simulink subsystem "dL2dz"  (R2024a)
settings: Solver=VariableStepAuto  StartTime=0.0  StopTime=10.0  RelTol=1e-3
undefined symbols (not defined in the file or in its folder): H, r
libraries: inductance x1
settings Model: Creator=Bocchio  LastModifiedBy=Bocchio

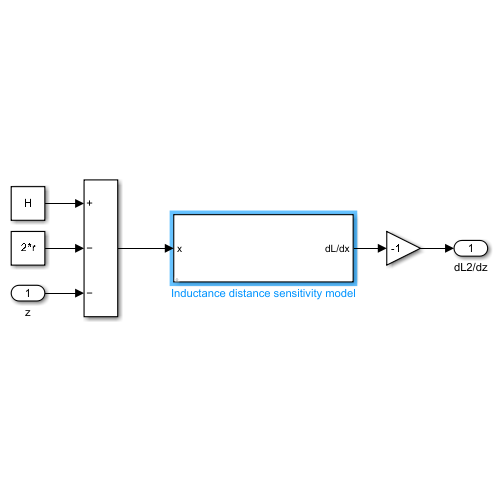
[thumbnail: Simulink's stored preview of the top-level diagram]
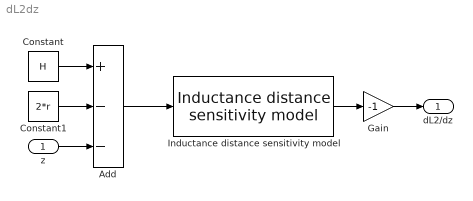
== system dL2dz ==
  z : Inport
  Add : Sum  Inputs=+--
  Constant : Constant  Value=H
  Constant1 : Constant  Value=2*r
  Gain : Gain  Gain=-1
  Inductance distance sensitivity model : inductance/Inductance distance sensitivity model  ax=a2z  Lx=L2z
  dL2/dz : Outport
  wires:
  Inductance distance sensitivity model/1 -> Gain/1
  Constant1/1 -> Add/2
  Constant/1 -> Add/1
  z/1 -> Add/3
  Add/1 -> Inductance distance sensitivity model/1
  Gain/1 -> dL2/dz/1
